simulink model "Antriebsstrangmodell_V2"  (R2019a)
settings: Solver=FixedStepAuto  StartTime=0.0  StopTime=t_Simulation  FixedStep=dt  RelTol=1e-3
undefined symbols (not defined in the file): alpha_Rotor, alpha_Stator, Anteil_Stator, cp_Luft, D_2a, delta, eta_EMaschine_Break_M_EMaschine, eta_EMaschine_Break_M_EMaschine_reku, eta_EMaschine_Break_n_EMaschine, eta_EMaschine_Break_n_EMaschine_reku, eta_EMaschine_Faktor_Volllast, eta_EMaschine_Table, eta_EMaschine_Table_reku, h_WC_pumpoff, h_WC_pumpon, lam_Luft, M_EMaschine_max, m_ER, m_RSL, m_RTO, m_RYO, m_SSL, m_STO, m_SYO, m_WH, nue_Luft, pump_start_limit, rho_Luft, share_EMaschine_Ummagnet_reku_Table, share_EMaschine_Ummagnet_Table, share_EMaschine_Wicklung_reku_Table, share_EMaschine_Wicklung_Table, share_EMaschine_WirkMech_reku_Table, share_EMaschine_WirkMech_Table, share_EMaschine_WirkZus_reku_Table, share_EMaschine_WirkZus_Table, T_Entwurf_Rotor, T_Entwurf_Stator, t_Simulation, T_Start_EMaschine, v_EC_corr, v_ER_corr, v_WH_corr, Verlustleistung_Fit
libraries: fl_lib x72, nesl_utility x26, SimscapeCustomBlocks_lib x8, simulink x3
(part 2 of 2)

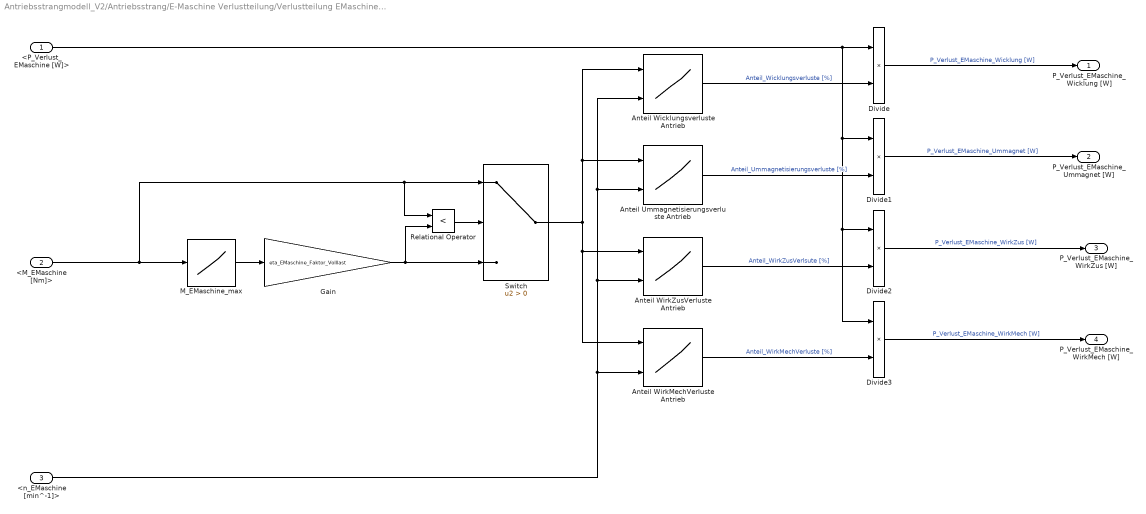
== system Antriebsstrangmodell_V2/Antriebsstrang/E-Maschine Verlustteilung/Verlustteilung EMaschine - Antrieb ==
  <P_Verlust_EMaschine [W]> : Inport
  <M_EMaschine [Nm]> : Inport  Port=2
  <n_EMaschine [min^-1]> : Inport  Port=3
  Anteil Ummagnetisierungsverluste Antrieb : Lookup_n-D  BreakpointsForDimension1=eta_EMaschine_Break_M_EMaschine  BreakpointsForDimension2=eta_EMaschine_Break_n_EMaschine  BeginIndexSearchUsingPreviousIndexResult=on  Table=share_EMaschine_Ummagnet_Table  ExtrapMethod=Clip  UseLastTableValue=on  InternalRulePriority=Speed  RndMeth=Simplest  InputSameDT=on
  Anteil Wicklungsverluste Antrieb : Lookup_n-D  BreakpointsForDimension1=eta_EMaschine_Break_M_EMaschine  BreakpointsForDimension2=eta_EMaschine_Break_n_EMaschine  BeginIndexSearchUsingPreviousIndexResult=on  Table=share_EMaschine_Wicklung_Table  ExtrapMethod=Clip  UseLastTableValue=on  InternalRulePriority=Speed  RndMeth=Simplest  InputSameDT=on
  Anteil WirkMechVerluste Antrieb : Lookup_n-D  BreakpointsForDimension1=eta_EMaschine_Break_M_EMaschine  BreakpointsForDimension2=eta_EMaschine_Break_n_EMaschine  BeginIndexSearchUsingPreviousIndexResult=on  Table=share_EMaschine_WirkMech_Table  ExtrapMethod=Clip  UseLastTableValue=on  InternalRulePriority=Speed  RndMeth=Simplest  InputSameDT=on
  Anteil WirkZusVerluste Antrieb : Lookup_n-D  BreakpointsForDimension1=eta_EMaschine_Break_M_EMaschine  BreakpointsForDimension2=eta_EMaschine_Break_n_EMaschine  BeginIndexSearchUsingPreviousIndexResult=on  Table=share_EMaschine_WirkZus_Table  ExtrapMethod=Clip  UseLastTableValue=on  InternalRulePriority=Speed  RndMeth=Simplest  InputSameDT=on
  Divide{,1..3} (4 alike) : Product  Inputs=**
  Gain : Gain  Gain=eta_EMaschine_Faktor_Volllast
  M_EMaschine_max : Lookup_n-D  NumberOfTableDimensions=1  BreakpointsForDimension1=M_EMaschine_max(1,:)  BeginIndexSearchUsingPreviousIndexResult=on  Table=M_EMaschine_max(2,:)  ExtrapMethod=Clip  UseLastTableValue=on  InternalRulePriority=Speed  RndMeth=Simplest  InputSameDT=on
  Relational Operator : RelationalOperator  Operator=<  OutDataTypeStr=boolean  RndMeth=Simplest
  Switch : Switch  Criteria=u2 > Threshold
  P_Verlust_EMaschine_Wicklung [W] : Outport
  P_Verlust_EMaschine_Ummagnet [W] : Outport  Port=2
  P_Verlust_EMaschine_WirkZus [W] : Outport  Port=3
  P_Verlust_EMaschine_WirkMech [W] : Outport  Port=4
  wires:
  Anteil Wicklungsverluste Antrieb/1 -> Divide/2  "Anteil_Wicklungsverluste [%]"
  M_EMaschine_max/1 -> Gain/1
  <n_EMaschine [min^-1]>/1 -> Anteil Wicklungsverluste Antrieb/2, Anteil Ummagnetisierungsverluste Antrieb/2, Anteil WirkZusVerluste Antrieb/2, Anteil WirkMechVerluste Antrieb/2
  <P_Verlust_EMaschine [W]>/1 -> Divide3/1, Divide2/1, Divide1/1, Divide/1
  Gain/1 -> Relational Operator/2, Switch/3
  Anteil WirkMechVerluste Antrieb/1 -> Divide3/2  "Anteil_WirkMechVerluste [%]"
  Switch/1 -> Anteil WirkMechVerluste Antrieb/1, Anteil WirkZusVerluste Antrieb/1, Anteil Wicklungsverluste Antrieb/1, Anteil Ummagnetisierungsverluste Antrieb/1
  Relational Operator/1 -> Switch/2
  Divide/1 -> P_Verlust_EMaschine_Wicklung [W]/1  "P_Verlust_EMaschine_Wicklung [W]"
  Anteil Ummagnetisierungsverluste Antrieb/1 -> Divide1/2  "Anteil_Ummagnetisierungsverluste [%]"
  Anteil WirkZusVerluste Antrieb/1 -> Divide2/2  "Anteil_WirkZusVerlsute [%]"
  Divide3/1 -> P_Verlust_EMaschine_WirkMech [W]/1  "P_Verlust_EMaschine_WirkMech [W]"
  Divide1/1 -> P_Verlust_EMaschine_Ummagnet [W]/1  "P_Verlust_EMaschine_Ummagnet [W]"
  Divide2/1 -> P_Verlust_EMaschine_WirkZus [W]/1  "P_Verlust_EMaschine_WirkZus [W]"
  <M_EMaschine [Nm]>/1 -> Relational Operator/1, Switch/1, M_EMaschine_max/1

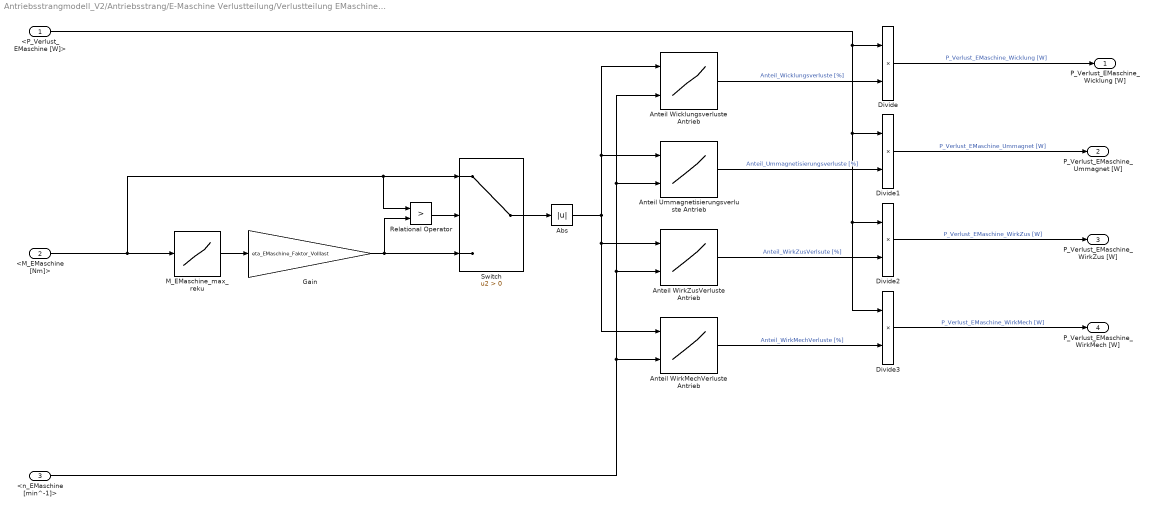
== system Antriebsstrangmodell_V2/Antriebsstrang/E-Maschine Verlustteilung/Verlustteilung EMaschine - Rekuperation ==
  <P_Verlust_EMaschine [W]> : Inport
  <M_EMaschine [Nm]> : Inport  Port=2
  <n_EMaschine [min^-1]> : Inport  Port=3
  Abs : Abs
  Anteil Ummagnetisierungsverluste Antrieb : Lookup_n-D  BreakpointsForDimension1=eta_EMaschine_Break_M_EMaschine  BreakpointsForDimension2=eta_EMaschine_Break_n_EMaschine  BeginIndexSearchUsingPreviousIndexResult=on  Table=share_EMaschine_Ummagnet_reku_Table  ExtrapMethod=Clip  UseLastTableValue=on  InternalRulePriority=Speed  RndMeth=Simplest  InputSameDT=on
  Anteil Wicklungsverluste Antrieb : Lookup_n-D  BreakpointsForDimension1=eta_EMaschine_Break_M_EMaschine  BreakpointsForDimension2=eta_EMaschine_Break_n_EMaschine  BeginIndexSearchUsingPreviousIndexResult=on  Table=share_EMaschine_Wicklung_reku_Table  ExtrapMethod=Clip  UseLastTableValue=on  InternalRulePriority=Speed  RndMeth=Simplest  InputSameDT=on
  Anteil WirkMechVerluste Antrieb : Lookup_n-D  BreakpointsForDimension1=eta_EMaschine_Break_M_EMaschine  BreakpointsForDimension2=eta_EMaschine_Break_n_EMaschine  BeginIndexSearchUsingPreviousIndexResult=on  Table=share_EMaschine_WirkMech_reku_Table  ExtrapMethod=Clip  UseLastTableValue=on  InternalRulePriority=Speed  RndMeth=Simplest  InputSameDT=on
  Anteil WirkZusVerluste Antrieb : Lookup_n-D  BreakpointsForDimension1=eta_EMaschine_Break_M_EMaschine  BreakpointsForDimension2=eta_EMaschine_Break_n_EMaschine  BeginIndexSearchUsingPreviousIndexResult=on  Table=share_EMaschine_WirkZus_reku_Table  ExtrapMethod=Clip  UseLastTableValue=on  InternalRulePriority=Speed  RndMeth=Simplest  InputSameDT=on
  Divide{,1..3} (4 alike) : Product  Inputs=**
  Gain : Gain  Gain=eta_EMaschine_Faktor_Volllast
  M_EMaschine_max_reku : Lookup_n-D  NumberOfTableDimensions=1  BreakpointsForDimension1=[-15,1700,2050,3400,4050,6100]  BeginIndexSearchUsingPreviousIndexResult=on  Table=[0.44,-52,-51,-37.5,-33,-27.25]  ExtrapMethod=Clip  UseLastTableValue=on  InternalRulePriority=Speed  RndMeth=Simplest  InputSameDT=on
  Relational Operator : RelationalOperator  Operator=>  OutDataTypeStr=boolean  RndMeth=Simplest
  Switch : Switch  Criteria=u2 > Threshold
  P_Verlust_EMaschine_Wicklung [W] : Outport
  P_Verlust_EMaschine_Ummagnet [W] : Outport  Port=2
  P_Verlust_EMaschine_WirkZus [W] : Outport  Port=3
  P_Verlust_EMaschine_WirkMech [W] : Outport  Port=4
  wires:
  Anteil Wicklungsverluste Antrieb/1 -> Divide/2  "Anteil_Wicklungsverluste [%]"
  M_EMaschine_max_reku/1 -> Gain/1
  <n_EMaschine [min^-1]>/1 -> Anteil Wicklungsverluste Antrieb/2, Anteil Ummagnetisierungsverluste Antrieb/2, Anteil WirkZusVerluste Antrieb/2, Anteil WirkMechVerluste Antrieb/2
  <P_Verlust_EMaschine [W]>/1 -> Divide3/1, Divide2/1, Divide1/1, Divide/1
  Gain/1 -> Relational Operator/2, Switch/3
  Anteil WirkMechVerluste Antrieb/1 -> Divide3/2  "Anteil_WirkMechVerluste [%]"
  Switch/1 -> Abs/1
  Relational Operator/1 -> Switch/2
  Divide/1 -> P_Verlust_EMaschine_Wicklung [W]/1  "P_Verlust_EMaschine_Wicklung [W]"
  Anteil Ummagnetisierungsverluste Antrieb/1 -> Divide1/2  "Anteil_Ummagnetisierungsverluste [%]"
  Anteil WirkZusVerluste Antrieb/1 -> Divide2/2  "Anteil_WirkZusVerlsute [%]"
  Divide3/1 -> P_Verlust_EMaschine_WirkMech [W]/1  "P_Verlust_EMaschine_WirkMech [W]"
  Divide1/1 -> P_Verlust_EMaschine_Ummagnet [W]/1  "P_Verlust_EMaschine_Ummagnet [W]"
  Divide2/1 -> P_Verlust_EMaschine_WirkZus [W]/1  "P_Verlust_EMaschine_WirkZus [W]"
  <M_EMaschine [Nm]>/1 -> M_EMaschine_max_reku/1, Relational Operator/1, Switch/1
  Abs/1 -> Anteil WirkMechVerluste Antrieb/1, Anteil WirkZusVerluste Antrieb/1, Anteil Wicklungsverluste Antrieb/1, Anteil Ummagnetisierungsverluste Antrieb/1

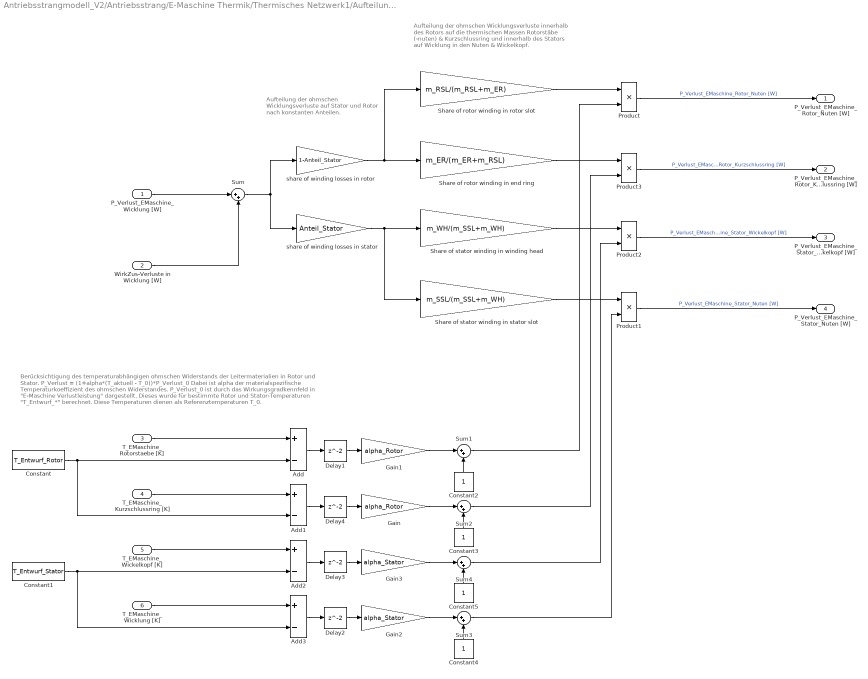
== system Antriebsstrangmodell_V2/Antriebsstrang/E-Maschine Thermik/Thermisches Netzwerk1/Aufteilung Wicklungsverluste + Temperaturabhängiger ohmscher Widerstand ==
  note: Berücksichtigung des temperaturabhängigen ohmschen Widerstands der Leitermaterialien in Rotor und Stator.
      | P_Verlust = (1+alpha*(T_aktuell - T_0))*P_Verlust_0
      | Dabei ist alpha der materialspezifische Temperaturkoeffizient des ohmschen Widerstandes.
      | P_Verlust_0 ist durch das Wirkungsgradkennfeld in "E-Maschine Verlustleistung" dargestellt. Dieses wurde für bestimmte Rotor und Stator-Temperaturen "T_Entwurf_*" berechnet. Diese Temperaturen dienen als Referenztemperaturen T_0.
  note: Aufteilung der ohmschen Wicklungsverluste innerhalb des Rotors auf die thermischen Massen Rotorstäbe (-nuten) & Kurzschlussring und innerhalb des Stators auf Wicklung in den Nuten & Wickelkopf.
  note: Aufteilung der ohmschen Wicklungsverluste auf Stator und Rotor nach konstanten Anteilen.
  P_Verlust_EMaschine_Wicklung [W] : Inport
  WirkZus-Verluste in Wicklung [W] : Inport  Port=2
  T_EMaschine_Rotorstaebe [K] : Inport  Port=3
  T_EMaschine_Kurzschlussring [K] : Inport  Port=4
  T_EMaschine_Wickelkopf [K] : Inport  Port=5
  T_EMaschine_Wicklung [K] : Inport  Port=6
  Add{,1..3} (4 alike) : Sum  Inputs=+-
  Constant : Constant  Value=T_Entwurf_Rotor
  Constant1 : Constant  Value=T_Entwurf_Stator
  Constant{2..5} (4 alike) : Constant
  Delay{1..4} (4 alike) : Delay
  Gain : Gain  Gain=alpha_Rotor
  Gain1 : Gain  Gain=alpha_Rotor
  Gain2 : Gain  Gain=alpha_Stator
  Gain3 : Gain  Gain=alpha_Stator
  Product{,1..3} (4 alike) : Product
  Share of rotor winding in end ring : Gain  Gain=m_ER/(m_ER+m_RSL)
  Share of rotor winding in rotor slot : Gain  Gain=m_RSL/(m_RSL+m_ER)
  Share of stator winding in stator slot : Gain  Gain=m_SSL/(m_SSL+m_WH)
  Share of stator winding in winding head : Gain  Gain=m_WH/(m_SSL+m_WH)
  Sum{,1..4} (5 alike) : Sum  Inputs=|++
  share of winding losses in rotor : Gain  Gain=1-Anteil_Stator
  share of winding losses in stator : Gain  Gain=Anteil_Stator
  P_Verlust_EMaschine_Rotor_Nuten [W] : Outport
  P_Verlust_EMaschine_Rotor_Kurzschlussring [W] : Outport  Port=2
  P_Verlust_EMaschine_Stator_Wickelkopf [W] : Outport  Port=3
  P_Verlust_EMaschine_Stator_Nuten [W] : Outport  Port=4
  wires:
  share of winding losses in stator/1 -> Share of stator winding in winding head/1, Share of stator winding in stator slot/1
  Sum/1 -> share of winding losses in stator/1, share of winding losses in rotor/1
  share of winding losses in rotor/1 -> Share of rotor winding in end ring/1, Share of rotor winding in rotor slot/1
  P_Verlust_EMaschine_Wicklung [W]/1 -> Sum/1
  WirkZus-Verluste in Wicklung [W]/1 -> Sum/2
  T_EMaschine_Rotorstaebe [K]/1 -> Add/1
  T_EMaschine_Wickelkopf [K]/1 -> Add2/1
  Constant1/1 -> Add3/2, Add2/2
  T_EMaschine_Wicklung [K]/1 -> Add3/1
  Add3/1 -> Delay2/1
  Add/1 -> Delay1/1
  Add1/1 -> Delay4/1
  Add2/1 -> Delay3/1
  Constant2/1 -> Sum1/2
  Constant3/1 -> Sum2/2
  Constant4/1 -> Sum3/2
  Constant5/1 -> Sum4/2
  Gain3/1 -> Sum4/1
  Gain2/1 -> Sum3/1
  Gain/1 -> Sum2/1
  Gain1/1 -> Sum1/1
  Share of rotor winding in rotor slot/1 -> Product/1
  Product/1 -> P_Verlust_EMaschine_Rotor_Nuten [W]/1  "P_Verlust_EMaschine_Rotor_Nuten [W]"
  Share of rotor winding in end ring/1 -> Product3/1
  Share of stator winding in winding head/1 -> Product2/1
  Share of stator winding in stator slot/1 -> Product1/1
  Sum1/1 -> Product/2
  Sum4/1 -> Product2/2
  Sum3/1 -> Product1/2
  Product3/1 -> P_Verlust_EMaschine_Rotor_Kurzschlussring [W]/1  "P_Verlust_EMaschine_Rotor_Kurzschlussring [W]"
  Product2/1 -> P_Verlust_EMaschine_Stator_Wickelkopf [W]/1  "P_Verlust_EMaschine_Stator_Wickelkopf [W]"
  Product1/1 -> P_Verlust_EMaschine_Stator_Nuten [W]/1  "P_Verlust_EMaschine_Stator_Nuten [W]"
  T_EMaschine_Kurzschlussring [K]/1 -> Add1/1
  Sum2/1 -> Product3/2
  Constant/1 -> Add/2, Add1/2
  Delay1/1 -> Gain1/1
  Delay4/1 -> Gain/1
  Delay3/1 -> Gain3/1
  Delay2/1 -> Gain2/1

== system Antriebsstrangmodell_V2/Antriebsstrang/E-Maschine Thermik/Thermisches Netzwerk1/Subsystem ==

== system Antriebsstrangmodell_V2/Antriebsstrang/E-Maschine Thermik/Thermisches Netzwerk1/Subsystem1 ==

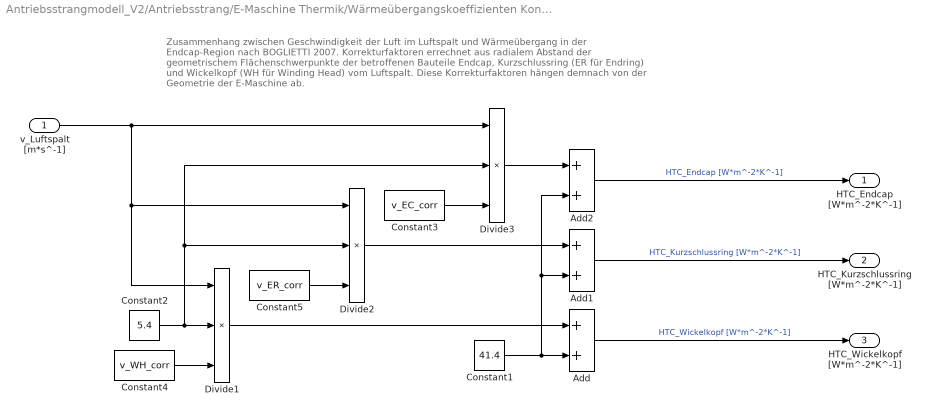
== system Antriebsstrangmodell_V2/Antriebsstrang/E-Maschine Thermik/Wärmeübergangskoeffizienten Konvektion Luftspalt und Endcap-Luft/Endcap-Luft-Konvektion ==
  note: Zusammenhang zwischen Geschwindigkeit der Luft im Luftspalt und Wärmeübergang in der Endcap-Region nach BOGLIETTI 2007.
      | Korrekturfaktoren errechnet aus radialem Abstand der geometrischem Flächenschwerpunkte der betroffenen Bauteile Endcap,
      | Kurzschlussring (ER für Endring) und Wickelkopf (WH für Winding Head) vom Luftspalt.
      | Diese Korrekturfaktoren hängen demnach von der Geometrie der E-Maschine ab.
  v_Luftspalt [m*s^-1] : Inport
  Add : Sum
  Add1 : Sum
  Add2 : Sum
  Constant1 : Constant  Value=41.4
  Constant2 : Constant  Value=5.4
  Constant3 : Constant  Value=v_EC_corr
  Constant4 : Constant  Value=v_WH_corr
  Constant5 : Constant  Value=v_ER_corr
  Divide1 : Product  Inputs=***
  Divide2 : Product  Inputs=***
  Divide3 : Product  Inputs=***
  HTC_Endcap [W*m^-2*K^-1] : Outport
  HTC_Kurzschlussring [W*m^-2*K^-1] : Outport  Port=2
  HTC_Wickelkopf [W*m^-2*K^-1] : Outport  Port=3
  wires:
  Add/1 -> HTC_Wickelkopf [W*m^-2*K^-1]/1  "HTC_Wickelkopf [W*m^-2*K^-1]"
  Constant3/1 -> Divide3/3
  Divide3/1 -> Add2/1
  v_Luftspalt [m*s^-1]/1 -> Divide1/1, Divide2/1, Divide3/1
  Constant2/1 -> Divide1/2, Divide3/2, Divide2/2
  Constant1/1 -> Add/2, Add1/2, Add2/2
  Constant4/1 -> Divide1/3
  Constant5/1 -> Divide2/3
  Divide2/1 -> Add1/1
  Divide1/1 -> Add/1
  Add1/1 -> HTC_Kurzschlussring [W*m^-2*K^-1]/1  "HTC_Kurzschlussring [W*m^-2*K^-1]"
  Add2/1 -> HTC_Endcap [W*m^-2*K^-1]/1  "HTC_Endcap [W*m^-2*K^-1]"

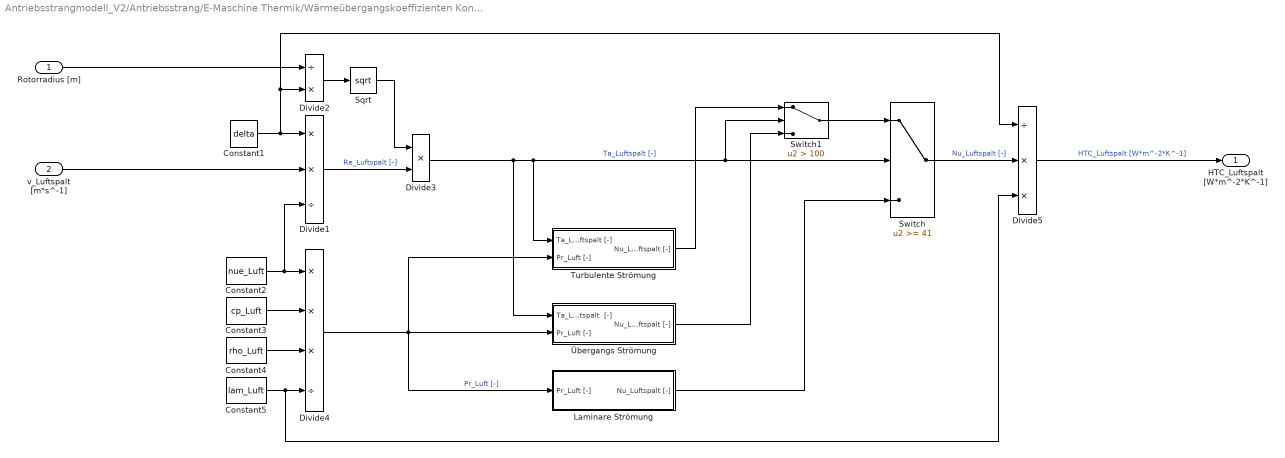
== system Antriebsstrangmodell_V2/Antriebsstrang/E-Maschine Thermik/Wärmeübergangskoeffizienten Konvektion Luftspalt und Endcap-Luft/Luftspalt-Konvektion ==
  Rotorradius [m] : Inport
  v_Luftspalt [m*s^-1] : Inport  Port=2
  Constant1 : Constant  Value=delta
  Constant2 : Constant  Value=nue_Luft
  Constant3 : Constant  Value=cp_Luft
  Constant4 : Constant  Value=rho_Luft
  Constant5 : Constant  Value=lam_Luft
  Divide1 : Product  Inputs=**/
  Divide2 : Product  Inputs=/*
  Divide3 : Product  Inputs=**
  Divide4 : Product  Inputs=***/
  Divide5 : Product  Inputs=/**
  Laminare Strömung : Subsystem
  Sqrt : Sqrt  SaturateOnIntegerOverflow=on
  Switch : Switch  Threshold=41
  Switch1 : Switch  Criteria=u2 > Threshold  Threshold=100
  Turbulente Strömung : Subsystem
  Übergangs Strömung : Subsystem
  HTC_Luftspalt [W*m^-2*K^-1] : Outport
  wires:
  Divide3/1 -> Switch1/2, Switch/2, Turbulente Strömung/1(Ta_Luftspalt [-]), Übergangs Strömung/1(Ta_Luftspalt  [-])  "Ta_Luftspalt [-]"
  Constant4/1 -> Divide4/3
  Divide4/1 -> Übergangs Strömung/2(Pr_Luft [-]), Laminare Strömung/1(Pr_Luft [-]), Turbulente Strömung/2(Pr_Luft [-])  "Pr_Luft [-]"
  Rotorradius [m]/1 -> Divide2/1
  Constant2/1 -> Divide1/3, Divide4/1
  Laminare Strömung/1(Nu_Luftspalt [-]) -> Switch/3
  Turbulente Strömung/1(Nu_Luftspalt [-]) -> Switch1/1
  Constant1/1 -> Divide5/1, Divide2/2, Divide1/1
  Übergangs Strömung/1(Nu_Luftspalt [-]) -> Switch1/3
  Constant5/1 -> Divide5/3, Divide4/4
  Divide1/1 -> Divide3/2  "Re_Luftspalt [-]"
  Switch1/1 -> Switch/1
  Switch/1 -> Divide5/2  "Nu_Luftspalt [-]"
  Sqrt/1 -> Divide3/1
  v_Luftspalt [m*s^-1]/1 -> Divide1/2
  Divide5/1 -> HTC_Luftspalt [W*m^-2*K^-1]/1  "HTC_Luftspalt [W*m^-2*K^-1]"
  Constant3/1 -> Divide4/2
  Divide2/1 -> Sqrt/1

== system Antriebsstrangmodell_V2/Antriebsstrang/E-Maschine Thermik/Wärmeübergangskoeffizienten Konvektion Luftspalt und Endcap-Luft/Luftspalt-Konvektion/Laminare Strömung ==
  Pr_Luft [-] : Inport
  Constant6 : Constant  Value=41
  Constant7 : Constant  Value=0.63
  Constant8 : Constant  Value=0.202
  Constant9 : Constant  Value=0.27
  Divide5 : Product  Inputs=***
  Math Function : Math  Operator=pow  SaturateOnIntegerOverflow=on
  Math Function1 : Math  Operator=pow  SaturateOnIntegerOverflow=on
  Nu_Luftspalt [-] : Outport
  wires:
  Constant6/1 -> Math Function/1
  Constant7/1 -> Math Function/2
  Math Function/1 -> Divide5/2
  Math Function1/1 -> Divide5/3
  Constant9/1 -> Math Function1/2
  Pr_Luft [-]/1 -> Math Function1/1
  Constant8/1 -> Divide5/1
  Divide5/1 -> Nu_Luftspalt [-]/1  "Nu_Luftspalt [-]"

== system Antriebsstrangmodell_V2/Antriebsstrang/E-Maschine Thermik/Wärmeübergangskoeffizienten Konvektion Luftspalt und Endcap-Luft/Luftspalt-Konvektion/Turbulente Strömung ==
  Ta_Luftspalt [-] : Inport
  Pr_Luft [-] : Inport  Port=2
  Constant7 : Constant  Value=0.5
  Constant8 : Constant  Value=0.386
  Constant9 : Constant  Value=0.27
  Divide5 : Product  Inputs=***
  Math Function : Math  Operator=pow  SaturateOnIntegerOverflow=on
  Math Function1 : Math  Operator=pow  SaturateOnIntegerOverflow=on
  Nu_Luftspalt [-] : Outport
  wires:
  Ta_Luftspalt [-]/1 -> Math Function/1
  Constant7/1 -> Math Function/2
  Math Function/1 -> Divide5/2
  Math Function1/1 -> Divide5/3
  Constant9/1 -> Math Function1/2
  Pr_Luft [-]/1 -> Math Function1/1
  Constant8/1 -> Divide5/1
  Divide5/1 -> Nu_Luftspalt [-]/1  "Nu_Luftspalt [-]"

== system Antriebsstrangmodell_V2/Antriebsstrang/E-Maschine Thermik/Wärmeübergangskoeffizienten Konvektion Luftspalt und Endcap-Luft/Luftspalt-Konvektion/Übergangs Strömung ==
  Ta_Luftspalt  [-] : Inport
  Pr_Luft [-] : Inport  Port=2
  Constant7 : Constant  Value=0.63
  Constant8 : Constant  Value=0.202
  Constant9 : Constant  Value=0.27
  Divide5 : Product  Inputs=***
  Math Function : Math  Operator=pow  SaturateOnIntegerOverflow=on
  Math Function1 : Math  Operator=pow  SaturateOnIntegerOverflow=on
  Nu_Luftspalt [-] : Outport
  wires:
  Ta_Luftspalt  [-]/1 -> Math Function/1
  Constant7/1 -> Math Function/2
  Math Function/1 -> Divide5/2
  Math Function1/1 -> Divide5/3
  Constant9/1 -> Math Function1/2
  Pr_Luft [-]/1 -> Math Function1/1
  Constant8/1 -> Divide5/1
  Divide5/1 -> Nu_Luftspalt [-]/1  "Nu_Luftspalt [-]"
